simulink model "z5_obserwator"  (R2021a)
settings: Solver=VariableStepAuto  StartTime=0.0  StopTime=10.0  RelTol=1e-3
values from neighbouring files (symbols this model uses):
  L1 = - (287708*so)/3465 - (79228*so^2)/3465 - (22628*so^3)/10395 - 1168108/10395    (= 3335.19499759)    [z6i7.m]
  L2 = (79228*so)/3465 + (22628*so^2)/3465 + (6448*so^3)/10395 + 287708/10395    (= -939.456661857)    [z6i7.m]
  L3 = - (22628*so)/3465 - (6448*so^2)/3465 - (1808*so^3)/10395 - 79228/10395    (= 258.646657047)    [z6i7.m]
  y = zeros(Ts + start, 1)    [DMC.m]    (also in PIDandDMC.m; z4odpskok.m = zeros(Ts, 1); z6stabilnosc.m = zeros(1,Ts + start); z_dod.m = out.simout4.signals.values)
settings Model: Creator=48604  LastModifiedBy=48604

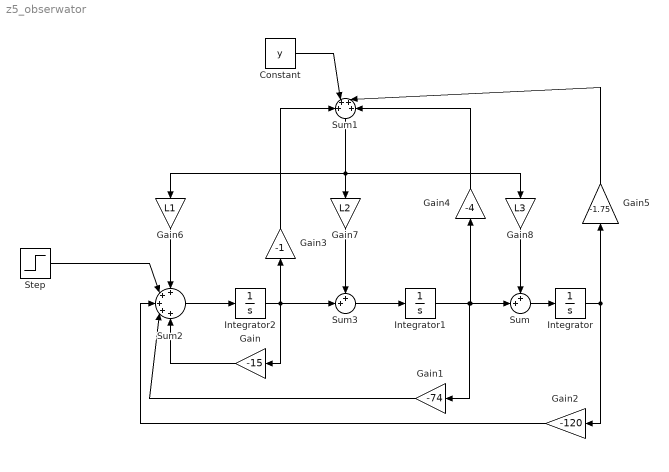
== system z5_obserwator ==
  Constant : Constant  Value=y
  Gain : Gain  Gain=-15
  Gain1 : Gain  Gain=-74
  Gain2 : Gain  Gain=-120
  Gain3 : Gain  Gain=-1
  Gain4 : Gain  Gain=-4
  Gain5 : Gain  Gain=-1.75
  Gain6 : Gain  Gain=L1
  Gain7 : Gain  Gain=L2
  Gain8 : Gain  Gain=L3
  Integrator : Integrator
  Integrator1 : Integrator
  Integrator2 : Integrator
  Step : Step  SampleTime=0
  Sum : Sum  Inputs=++|
  Sum1 : Sum  Inputs=++++
  Sum2 : Sum  Inputs=+++++
  Sum3 : Sum  Inputs=++|
  wires:
  Integrator1/1 -> Gain4/1, Sum/2, Gain1/1
  Integrator2/1 -> Sum3/2, Gain3/1, Gain/1
  Sum2/1 -> Integrator2/1
  Gain/1 -> Sum2/5
  Gain1/1 -> Sum2/4
  Integrator/1 -> Gain5/1, Gain2/1
  Gain2/1 -> Sum2/3
  Step/1 -> Sum2/2
  Constant/1 -> Sum1/2
  Gain3/1 -> Sum1/1
  Gain4/1 -> Sum1/4
  Gain5/1 -> Sum1/3
  Sum/1 -> Integrator/1
  Sum3/1 -> Integrator1/1
  Gain8/1 -> Sum/1
  Gain7/1 -> Sum3/1
  Gain6/1 -> Sum2/1
  Sum1/1 -> Gain8/1, Gain7/1, Gain6/1
